simulink model "HeadwayControlSimplified-DESKTOP-J3FI8VF"  (R2018a)
settings: Solver=ode45  StartTime=0.0  StopTime=tsim  MaxStep=.1  RelTol=1e-3
values from neighbouring files (symbols this model uses):
  EndVel = (Time2-Time1)*Slope+StartVel    (= 31.525)    [HeadwayControlSimScript.m]    (also in HeadwayControlSimScriptExperiment.m; HeadwayControlSimScriptSimplified.m)
  h = 2    [HeadwayControlSimScript.m]    (also in HeadwayControlSimScriptExperiment.m; HeadwayControlSimScriptSimplified.m)
  InputNum = 3    [HeadwayControlSimScript.m]    (also in HeadwayControlSimScriptExperiment.m; HeadwayControlSimScriptSimplified.m)
  InputTime = 1    [HeadwayControlSimScript.m]    (also in HeadwayControlSimScriptExperiment.m; HeadwayControlSimScriptSimplified.m)
  lambda = 0.001    [HeadwayControlSimScript.m]    (also in HeadwayControlSimScriptExperiment.m = 0.135; HeadwayControlSimScriptSimplified.m)
  Slope = 0.5*g    (= 4.905)    [HeadwayControlSimScript.m]    (also in HeadwayControlSimScriptExperiment.m; HeadwayControlSimScriptSimplified.m)
  StartVel = 7    [HeadwayControlSimScript.m]    (also in HeadwayControlSimScriptExperiment.m; HeadwayControlSimScriptSimplified.m)
  tau = .5    (= 0.5)    [HeadwayControlSimScript.m]    (also in HeadwayControlSimScriptExperiment.m; HeadwayControlSimScriptSimplified.m)
libraries: simulink x2
settings Model: Creator=domin  LastModifiedBy=domin

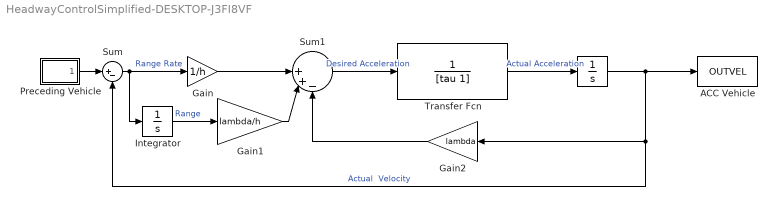
== system HeadwayControlSimplified-DESKTOP-J3FI8VF ==
  " " : Integrator  InitialCondition=StartVel
  ACC Vehicle : ToWorkspace  VariableName=OUTVEL  SampleTime=-1
  Gain : Gain  Gain=1/h
  Gain1 : Gain  Gain=lambda/h
  Gain2 : Gain  Gain=lambda
  Integrator : Integrator  InitialCondition=h*StartVel
  Preceding Vehicle : Subsystem
  Sum : Sum  Inputs=|+-
  Sum1 : Sum  Inputs=||++-
  Transfer Fcn : TransferFcn  Denominator=[tau 1]
  wires:
  Sum/1 -> Integrator/1, Gain/1  "Range Rate"
  Integrator/1 -> Gain1/1  "Range"
  Gain/1 -> Sum1/1
  Gain1/1 -> Sum1/2
  Sum1/1 -> Transfer Fcn/1  "Desired Acceleration"
  Transfer Fcn/1 -> " "/1  "Actual Acceleration"
  " "/1 -> ACC Vehicle/1, Sum/2, Gain2/1  "Actual  Velocity"
  Gain2/1 -> Sum1/3
  Preceding Vehicle/1(INVEL) -> Sum/1

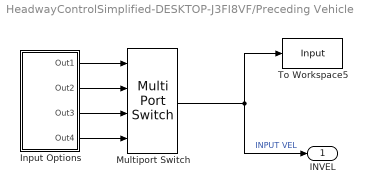
== system HeadwayControlSimplified-DESKTOP-J3FI8VF/Preceding Vehicle ==
  Input Options : Subsystem
  Multiport Switch : MultiPortSwitch
  To Workspace5 : ToWorkspace  VariableName=Input  SampleTime=-1
  INVEL : Outport
  wires:
  Multiport Switch/1 -> INVEL/1, To Workspace5/1  "INPUT VEL"
  Input Options/4(Out4) -> Multiport Switch/4
  Input Options/1(Out1) -> Multiport Switch/1
  Input Options/3(Out3) -> Multiport Switch/3
  Input Options/2(Out2) -> Multiport Switch/2

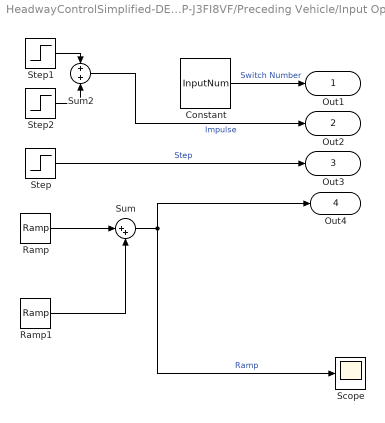
== system HeadwayControlSimplified-DESKTOP-J3FI8VF/Preceding Vehicle/Input Options ==
  Constant : Constant  Value=InputNum
  Ramp : simulink/Sources/Ramp  slope=Slope  start=Time1  InitialOutput=StartVel
  Ramp1 : simulink/Sources/Ramp  slope=-Slope  start=Time2  InitialOutput=0
  Scope : Scope
  Step : Step  Time=InputTime  Before=StartVel  After=EndVel  SampleTime=0
  Step1 : Step  Time=InputTime  Before=StartVel  After=StartVel+(1*10^10)  SampleTime=0
  Step2 : Step  Time=InputTime + (1*10^-10)  After=-(1*10^10)  SampleTime=0
  Sum : Sum  Inputs=|++
  Sum2 : Sum
  Out1 : Outport
  Out2 : Outport  Port=2
  Out3 : Outport  Port=3
  Out4 : Outport  Port=4
  wires:
  Sum2/1 -> Out2/1  "Impulse"
  Constant/1 -> Out1/1  "Switch Number"
  Step2/1 -> Sum2/2
  Step1/1 -> Sum2/1
  Step/1 -> Out3/1  "Step"
  Ramp/1 -> Sum/1
  Ramp1/1 -> Sum/2
  Sum/1 -> Out4/1, Scope/1  "Ramp"
